simulink model "cpu_time_test"  (R2014b)
settings: Solver=FixedStepDiscrete  StartTime=0.0  StopTime=inf  FixedStep=0.0001  RelTol=1e-3
settings Model: Creator=wangsp1  LastModifiedBy=wangsp1

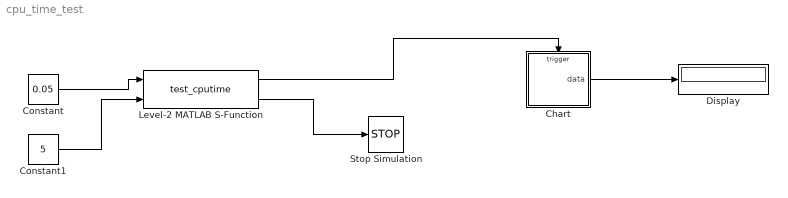
== system cpu_time_test ==
  Chart : Stateflow chart  TreatAsAtomicUnit=on
  Constant : Constant  Value=0.05
  Constant1 : Constant  Value=5
  Display : Display
  Level-2 MATLAB S-Function : M-S-Function  FunctionName=test_cputime
  Stop Simulation : Stop
  wires:
  Constant/1 -> Level-2 MATLAB S-Function/1
  Level-2 MATLAB S-Function/1 -> Chart/Trigger
  Constant1/1 -> Level-2 MATLAB S-Function/2
  Level-2 MATLAB S-Function/2 -> Stop Simulation/1
  Chart/1(data) -> Display/1

== stateflow chart cpu_time_test/Chart ==
  state s1
  state s2
  (default) -> s1 : {data=0;}
  s1 -> s2 : {data++;}
  s2 -> s1 : {data++;}
  data: data output double
  events: event input RISING_EDGE_EVENT
